simulink model "W04_7_ssa_test"  (R2024b)
settings: Solver=ode4  StartTime=0.0  StopTime=1080  FixedStep=0.05  RelTol=1e-3
settings Model: Creator=admin  LastModifiedBy=admin

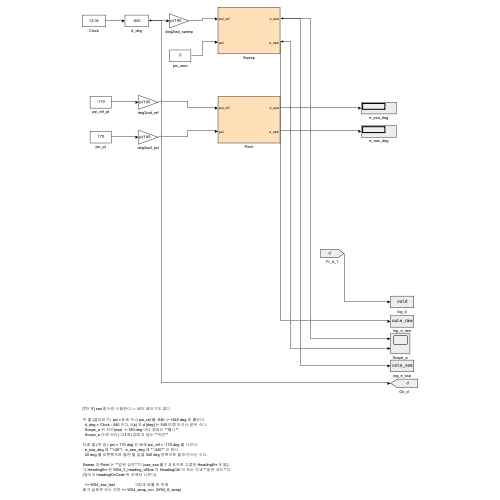
[thumbnail: Simulink's stored preview of the top-level diagram]
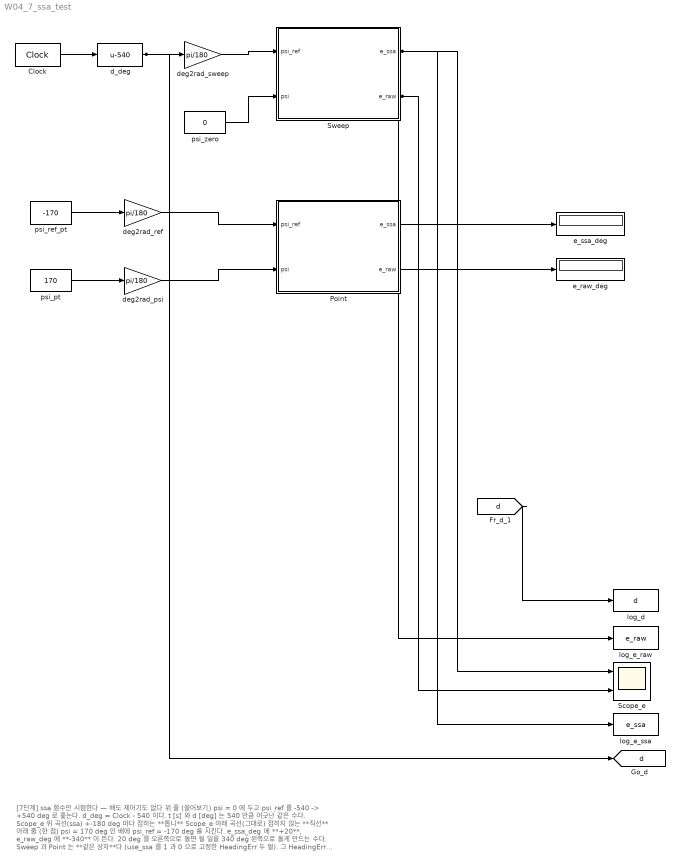
== system W04_7_ssa_test ==
  note: [7단계] ssa 함수만 시험한다 — 배도 제어기도 없다
      |
      | 위 줄 (쓸어보기)  psi = 0 에 두고 psi_ref 를 -540 -> +540 deg 로 훑는다.
      |   d_deg = Clock - 540 이다. t [s] 와 d [deg] 는 540 만큼 어긋난 같은 수다.
      |   Scope_e 위 곡선(ssa)  +-180 deg 마다 접히는 **톱니**
      |   Scope_e 아래 곡선(그대로) 접히지 않는 **직선**
      |
      | 아래 줄 (한 점)  psi = 170 deg 인 배에 psi_ref = -170 deg 를 시킨다.
      |   e_ssa_deg 에 **+20**,  e_raw_deg 에 **-340** 이 뜬다.
      |   20 deg 를 오른쪽으로 돌면 될 일을 340 deg 왼쪽으로 돌게 만드는 수다.
      |
      | Sweep 과 Point 는 **같은 상자**다 (use_ssa 를 1 과 0 으로 고정한 HeadingErr 두 벌).
      | 그 HeadingErr 은 W04_3_heading_offline 의 HeadingCtrl 이 쓰는 것과 **같은 코드**다
      | (빌더의 headingErrCode 한 곳에서 나온다).
      |
      |   >> W04_ssa_test                  그림과 표를 한 번에
      | 배가 실제로 도는 것은 >> W04_wrap_run  (W04_6_wrap)
  Clock : DigitalClock  SampleTime=0.05
  Point : Subsystem
  Scope_e : Scope  NumInputPorts=2
  Sweep : Subsystem
  d_deg : Bias  Bias=-540  SaturateOnIntegerOverflow=off
  deg2rad_psi : Gain  Gain=pi/180
  deg2rad_ref : Gain  Gain=pi/180
  deg2rad_sweep : Gain  Gain=pi/180
  e_raw_deg : Display
  e_ssa_deg : Display
  log_d : ToWorkspace  VariableName=d  SaveFormat=Timeseries  SampleTime=0.05
  log_e_raw : ToWorkspace  VariableName=e_raw  SaveFormat=Timeseries  SampleTime=0.05
  log_e_ssa : ToWorkspace  VariableName=e_ssa  SaveFormat=Timeseries  SampleTime=0.05
  psi_pt : Constant  Value=170
  psi_ref_pt : Constant  Value=-170
  psi_zero : Constant  Value=0
  tag scope: d=global
  wires:
  Clock/1 -> d_deg/1
  deg2rad_sweep/1 -> Sweep/1(psi_ref)
  psi_zero/1 -> Sweep/2(psi)
  psi_ref_pt/1 -> deg2rad_ref/1
  psi_pt/1 -> deg2rad_psi/1
  deg2rad_ref/1 -> Point/1(psi_ref)
  deg2rad_psi/1 -> Point/2(psi)
  Point/1(e_ssa) -> e_ssa_deg/1
  Point/2(e_raw) -> e_raw_deg/1
  [d] -> log_d/1
  Sweep/2(e_raw) -> log_e_raw/1, Scope_e/2
  Sweep/1(e_ssa) -> log_e_ssa/1, Scope_e/1
  d_deg/1 -> [d], deg2rad_sweep/1

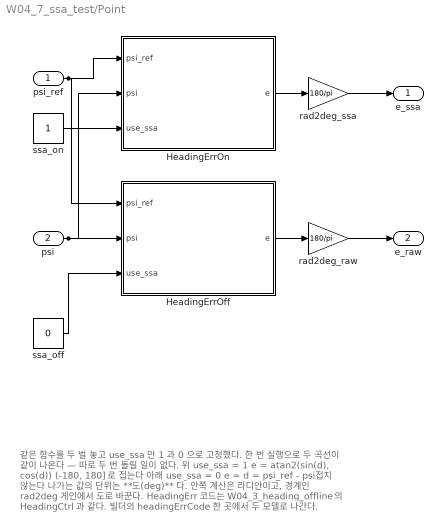
== system W04_7_ssa_test/Point ==
  note: 같은 함수를 두 벌 놓고 use_ssa 만 1 과 0 으로 고정했다.
      | 한 번 실행으로 두 곡선이 같이 나온다 — 따로 두 번 돌릴 일이 없다.
      |
      |   위  use_ssa = 1   e = atan2(sin(d), cos(d))   (-180, 180] 로 접는다
      |   아래 use_ssa = 0   e = d = psi_ref - psi       접지 않는다
      |
      | 나가는 값의 단위는 **도(deg)** 다. 안쪽 계산은 라디안이고,
      | 경계인 rad2deg 게인에서 도로 바꾼다.
      |
      | HeadingErr 코드는 W04_3_heading_offline 의 HeadingCtrl 과 같다.
      | 빌더의 headingErrCode 한 곳에서 두 모델로 나간다.
  psi_ref : Inport
  psi : Inport  Port=2
  HeadingErrOff : MATLAB Function  TreatAsAtomicUnit=on
  HeadingErrOn : MATLAB Function  TreatAsAtomicUnit=on
  rad2deg_raw : Gain  Gain=180/pi
  rad2deg_ssa : Gain  Gain=180/pi
  ssa_off : Constant  Value=0
  ssa_on : Constant
  e_ssa : Outport
  e_raw : Outport  Port=2
  wires:
  HeadingErrOff/1(e) -> rad2deg_raw/1
  ssa_on/1 -> HeadingErrOn/3(use_ssa)
  psi_ref/1 -> HeadingErrOn/1(psi_ref), HeadingErrOff/1(psi_ref)
  psi/1 -> HeadingErrOn/2(psi), HeadingErrOff/2(psi)
  ssa_off/1 -> HeadingErrOff/3(use_ssa)
  HeadingErrOn/1(e) -> rad2deg_ssa/1
  rad2deg_ssa/1 -> e_ssa/1
  rad2deg_raw/1 -> e_raw/1

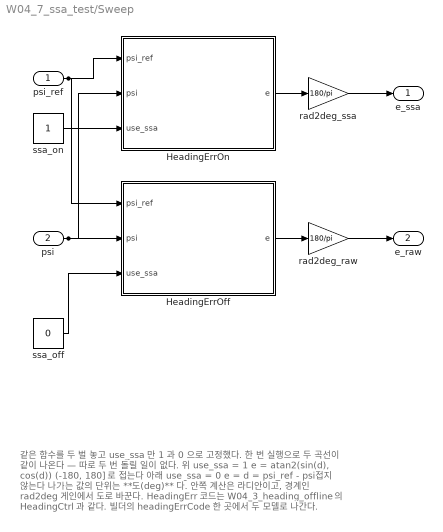
== system W04_7_ssa_test/Sweep ==
  note: 같은 함수를 두 벌 놓고 use_ssa 만 1 과 0 으로 고정했다.
      | 한 번 실행으로 두 곡선이 같이 나온다 — 따로 두 번 돌릴 일이 없다.
      |
      |   위  use_ssa = 1   e = atan2(sin(d), cos(d))   (-180, 180] 로 접는다
      |   아래 use_ssa = 0   e = d = psi_ref - psi       접지 않는다
      |
      | 나가는 값의 단위는 **도(deg)** 다. 안쪽 계산은 라디안이고,
      | 경계인 rad2deg 게인에서 도로 바꾼다.
      |
      | HeadingErr 코드는 W04_3_heading_offline 의 HeadingCtrl 과 같다.
      | 빌더의 headingErrCode 한 곳에서 두 모델로 나간다.
  psi_ref : Inport
  psi : Inport  Port=2
  HeadingErrOff : MATLAB Function  TreatAsAtomicUnit=on
  HeadingErrOn : MATLAB Function  TreatAsAtomicUnit=on
  rad2deg_raw : Gain  Gain=180/pi
  rad2deg_ssa : Gain  Gain=180/pi
  ssa_off : Constant  Value=0
  ssa_on : Constant
  e_ssa : Outport
  e_raw : Outport  Port=2
  wires:
  psi_ref/1 -> HeadingErrOn/1(psi_ref), HeadingErrOff/1(psi_ref)
  ssa_on/1 -> HeadingErrOn/3(use_ssa)
  psi/1 -> HeadingErrOn/2(psi), HeadingErrOff/2(psi)
  ssa_off/1 -> HeadingErrOff/3(use_ssa)
  rad2deg_ssa/1 -> e_ssa/1
  HeadingErrOff/1(e) -> rad2deg_raw/1
  HeadingErrOn/1(e) -> rad2deg_ssa/1
  rad2deg_raw/1 -> e_raw/1

== matlab function W04_7_ssa_test/Sweep/HeadingErrOn ==
  data: psi_ref input; e output; psi input; use_ssa input
function e = HeadingErr(psi_ref, psi, use_ssa)
%#codegen
% Heading error [rad].
d = psi_ref - psi;
if use_ssa >= 0.5
    % ssa : shortest signed angle, wrapped to (-pi, pi]
    e = atan2(sin(d), cos(d));
else
    % no wrap : 170 deg -> -170 deg becomes -340 deg, not +20 deg
    e = d;
end

== matlab function W04_7_ssa_test/Point/HeadingErrOn ==
  data: psi_ref input; e output; psi input; use_ssa input
function e = HeadingErr(psi_ref, psi, use_ssa)
%#codegen
% Heading error [rad].
d = psi_ref - psi;
if use_ssa >= 0.5
    % ssa : shortest signed angle, wrapped to (-pi, pi]
    e = atan2(sin(d), cos(d));
else
    % no wrap : 170 deg -> -170 deg becomes -340 deg, not +20 deg
    e = d;
end

== matlab function W04_7_ssa_test/Point/HeadingErrOff ==
  data: psi_ref input; e output; psi input; use_ssa input
function e = HeadingErr(psi_ref, psi, use_ssa)
%#codegen
% Heading error [rad].
d = psi_ref - psi;
if use_ssa >= 0.5
    % ssa : shortest signed angle, wrapped to (-pi, pi]
    e = atan2(sin(d), cos(d));
else
    % no wrap : 170 deg -> -170 deg becomes -340 deg, not +20 deg
    e = d;
end

== matlab function W04_7_ssa_test/Sweep/HeadingErrOff ==
  data: psi_ref input; e output; psi input; use_ssa input
function e = HeadingErr(psi_ref, psi, use_ssa)
%#codegen
% Heading error [rad].
d = psi_ref - psi;
if use_ssa >= 0.5
    % ssa : shortest signed angle, wrapped to (-pi, pi]
    e = atan2(sin(d), cos(d));
else
    % no wrap : 170 deg -> -170 deg becomes -340 deg, not +20 deg
    e = d;
end
